simulink model "GuytonModel1972WithSubsystems_R2018_new"  (Simulink 9.1)
settings: Solver=ode23tb  StartTime=0.0  StopTime=inf  RelTol=1e-3  EnableMultiTasking=on
(part 3 of 3)

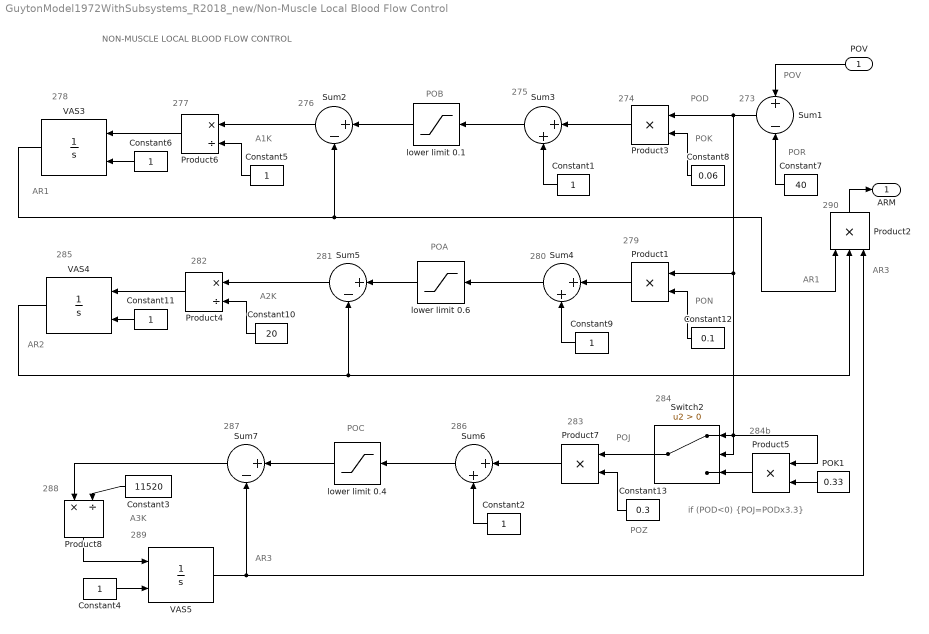
== system GuytonModel1972WithSubsystems_R2018_new/Non-Muscle Local Blood Flow Control  ==
  note: 273
  note: 285
  note: 281
  note: 280
  note: 279
  note: 290
  note: 286
  note: AR2
  note: AR1
  note: 287
  note: AR3
  note: POV
  note: 284b
  note: A2K
  note: POC
  note: AR1
  note: POZ
  note: 284
  note: PON
  note: 288
  note: POR
  note: POJ
  note: 289
  note: POK
  note: POA
  note: NON-MUSCLE LOCAL BLOOD FLOW CONTROL
  note: 278
  note: if (POD<0) {POJ=PODx3.3}
  note: A3K
  note: 282
  note: AR3
  note: 277
  note: 283
  note: 276
  note: 275
  note: POB
  note: 274
  note: A1K
  note: POD
  POV : Inport
  " VAS3" : Integrator  InitialConditionSource=external
  " VAS4" : Integrator  InitialConditionSource=external
  " VAS5" : Integrator  InitialConditionSource=external
  Constant{1..2,4..6,9,11} (7 alike) : Constant
  Constant10 : Constant  Value=20
  Constant12 : Constant  Value=0.1
  Constant13 : Constant  Value=0.3
  Constant3 : Constant  Value=11520
  Constant7 : Constant  Value=40
  Constant8 : Constant  Value=0.06
  POK1 : Constant  Value=0.33
  Product{1,3,5,7} (4 alike) : Product  SaturateOnIntegerOverflow=on  RndMeth=Zero  InputSameDT=on  OutDataTypeStr=Inherit: Same as first input
  Product2 : Product  Inputs=3  SaturateOnIntegerOverflow=on  RndMeth=Zero  InputSameDT=on  OutDataTypeStr=Inherit: Same as first input
  Product4 : Product  Inputs=*/  SaturateOnIntegerOverflow=on  RndMeth=Zero  InputSameDT=on  OutDataTypeStr=Inherit: Same as first input
  Product6 : Product  Inputs=*/  SaturateOnIntegerOverflow=on  RndMeth=Zero  InputSameDT=on  OutDataTypeStr=Inherit: Same as first input
  Product8 : Product  Inputs=*/  SaturateOnIntegerOverflow=on  RndMeth=Zero  InputSameDT=on  OutDataTypeStr=Inherit: Same as first input
  Sum1 : Sum  Inputs=+|-  SaturateOnIntegerOverflow=on  InputSameDT=on  OutDataTypeStr=Inherit: Same as first input
  Sum2 : Sum  Inputs=|+-  SaturateOnIntegerOverflow=on  InputSameDT=on  OutDataTypeStr=Inherit: Same as first input
  Sum3 : Sum  Inputs=|++  SaturateOnIntegerOverflow=on  InputSameDT=on  OutDataTypeStr=Inherit: Same as first input
  Sum4 : Sum  Inputs=|++  SaturateOnIntegerOverflow=on  InputSameDT=on  OutDataTypeStr=Inherit: Same as first input
  Sum5 : Sum  Inputs=|+-  SaturateOnIntegerOverflow=on  InputSameDT=on  OutDataTypeStr=Inherit: Same as first input
  Sum6 : Sum  Inputs=|++  SaturateOnIntegerOverflow=on  InputSameDT=on  OutDataTypeStr=Inherit: Same as first input
  Sum7 : Sum  Inputs=|+-  SaturateOnIntegerOverflow=on  InputSameDT=on  OutDataTypeStr=Inherit: Same as first input
  Switch2 : Switch  Criteria=u2 > Threshold  SaturateOnIntegerOverflow=on  InputSameDT=on
  lower limit 0.1 : Saturate  UpperLimit=inf  LowerLimit=0.2  LinearizeAsGain=off
  lower limit 0.4 : Saturate  UpperLimit=inf  LowerLimit=0.3  LinearizeAsGain=off
  lower limit 0.6 : Saturate  UpperLimit=inf  LowerLimit=0.5  LinearizeAsGain=off
  ARM : Outport
  wires:
  Product2/1 -> ARM/1
  Product7/1 -> Sum6/1
  " VAS3"/1 -> Sum2/2, Product2/1
  lower limit 0.1/1 -> Sum2/1
  Constant3/1 -> Product8/2
  Constant5/1 -> Product6/2
  Product3/1 -> Sum3/1
  Product5/1 -> Switch2/3
  Sum7/1 -> Product8/1
  Product1/1 -> Sum4/1
  POV/1 -> Sum1/1
  " VAS4"/1 -> Sum5/2, Product2/2
  Constant11/1 -> " VAS4"/2
  Constant8/1 -> Product3/2
  Constant10/1 -> Product4/2
  Sum3/1 -> lower limit 0.1/1
  Constant4/1 -> " VAS5"/2
  Product8/1 -> " VAS5"/1
  Product4/1 -> " VAS4"/1
  " VAS5"/1 -> Sum7/2, Product2/3
  POK1/1 -> Product5/2
  Constant6/1 -> " VAS3"/2
  lower limit 0.6/1 -> Sum5/1
  Sum6/1 -> lower limit 0.4/1
  Constant2/1 -> Sum6/2
  Sum5/1 -> Product4/1
  lower limit 0.4/1 -> Sum7/1
  Sum4/1 -> lower limit 0.6/1
  Constant12/1 -> Product1/2
  Constant1/1 -> Sum3/2
  Switch2/1 -> Product7/1
  Constant9/1 -> Sum4/2
  Product6/1 -> " VAS3"/1
  Sum1/1 -> Product3/1, Product1/1, Switch2/1, Product5/1, Switch2/2
  Constant13/1 -> Product7/2
  Sum2/1 -> Product6/1
  Constant7/1 -> Sum1/2

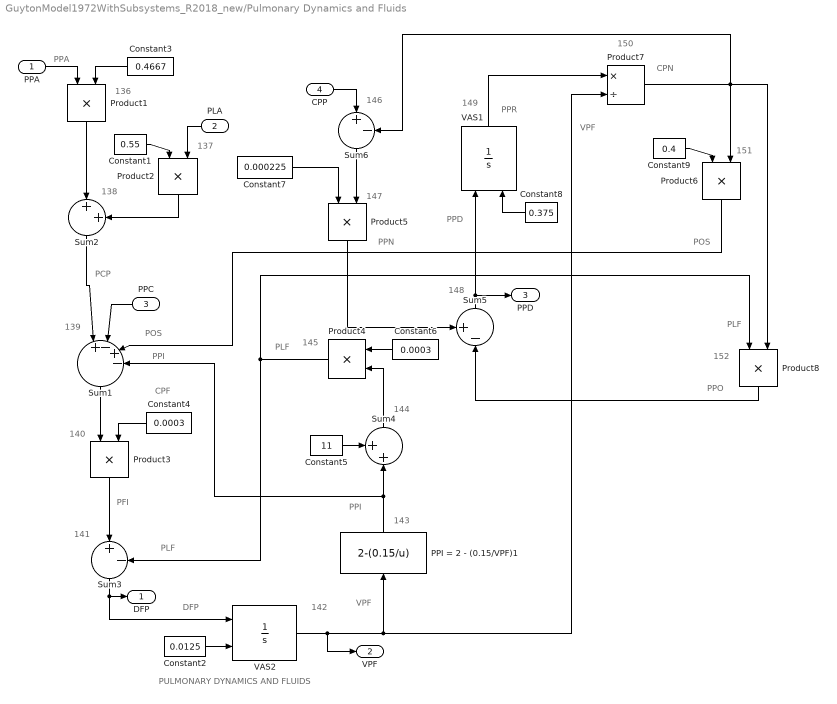
== system GuytonModel1972WithSubsystems_R2018_new/Pulmonary Dynamics and Fluids ==
  note: PULMONARY DYNAMICS AND FLUIDS
  note: 152
  note: 149
  note: 151
  note: POS
  note: DFP
  note: PPR
  note: CPF
  note: PLF
  note: VPF
  note: CPN
  note: VPF
  note: 136
  note: 147
  note: PPN
  note: 137
  note: POS
  note: PPI
  note: PPO
  note: PPD
  note: PLF
  note: PPA
  note: 141
  note: PLF
  note: PCP
  note: 138
  note: 148
  note: PFI
  note: 140
  note: 142
  note: 139
  note: 144
  note: 146
  note: 150
  note: PPI
  note: 143
  note: 145
  PPA : Inport
  PLA : Inport  Port=2
  PPC : Inport  Port=3
  CPP : Inport  Port=4
  " VAS1" : Integrator  InitialConditionSource=external
  " VAS2" : Integrator  InitialConditionSource=external
  Constant1 : Constant  Value=0.55
  Constant2 : Constant  Value=0.0125
  Constant3 : Constant  Value=0.4667
  Constant4 : Constant  Value=0.0003
  Constant5 : Constant  Value=11
  Constant6 : Constant  Value=0.0003
  Constant7 : Constant  Value=0.000225
  Constant8 : Constant  Value=0.375
  Constant9 : Constant  Value=0.4
  PPI = 2 - (0.15/VPF)1 : Fcn  Expr=2-(0.15/u)
  Product{1..6,8} (7 alike) : Product  SaturateOnIntegerOverflow=on  RndMeth=Zero  InputSameDT=on  OutDataTypeStr=Inherit: Same as first input
  Product7 : Product  Inputs=*/  SaturateOnIntegerOverflow=on  RndMeth=Zero  InputSameDT=on  OutDataTypeStr=Inherit: Same as first input
  Sum1 : Sum  Inputs=||+-+-  SaturateOnIntegerOverflow=on  InputSameDT=on  OutDataTypeStr=Inherit: Same as first input
  Sum2 : Sum  Inputs=|++  SaturateOnIntegerOverflow=on  InputSameDT=on  OutDataTypeStr=Inherit: Same as first input
  Sum3 : Sum  Inputs=|+-  SaturateOnIntegerOverflow=on  InputSameDT=on  OutDataTypeStr=Inherit: Same as first input
  Sum4 : Sum  Inputs=++|  SaturateOnIntegerOverflow=on  InputSameDT=on  OutDataTypeStr=Inherit: Same as first input
  Sum5 : Sum  Inputs=+-|  SaturateOnIntegerOverflow=on  InputSameDT=on  OutDataTypeStr=Inherit: Same as first input
  Sum6 : Sum  Inputs=|+-  SaturateOnIntegerOverflow=on  InputSameDT=on  OutDataTypeStr=Inherit: Same as first input
  DFP : Outport
  VPF : Outport  Port=2
  PPD : Outport  Port=3
  wires:
  Constant2/1 -> " VAS2"/2
  Constant3/1 -> Product1/2
  Sum4/1 -> Product4/2
  Sum6/1 -> Product5/2
  Product4/1 -> Product8/1, Sum3/2
  PLA/1 -> Product2/2
  Sum5/1 -> " VAS1"/1, PPD/1
  Constant7/1 -> Product5/1
  Product8/1 -> Sum5/2
  Product5/1 -> Sum5/1
  Sum1/1 -> Product3/1
  Sum2/1 -> Sum1/1
  PPI = 2 - (0.15/VPF)1/1 -> Sum1/4, Sum4/2
  " VAS2"/1 -> VPF/1, PPI = 2 - (0.15/VPF)1/1, Product7/2
  Product6/1 -> Sum1/3
  Constant4/1 -> Product3/2
  Constant6/1 -> Product4/1
  Sum3/1 -> DFP/1, " VAS2"/1
  Constant5/1 -> Sum4/1
  Constant9/1 -> Product6/1
  Product1/1 -> Sum2/1
  PPA/1 -> Product1/1
  Constant1/1 -> Product2/1
  Constant8/1 -> " VAS1"/2
  Product2/1 -> Sum2/2
  " VAS1"/1 -> Product7/1
  Product7/1 -> Product6/2, Sum6/2, Product8/2
  Product3/1 -> Sum3/1
  CPP/1 -> Sum6/1
  PPC/1 -> Sum1/2

== system GuytonModel1972WithSubsystems_R2018_new/Red Cells And Viscosity ==
  note: HKM
  note: 336
  note: HMK
  note: HM
  note: 336b
  note: VIB
  note: HM2
  note: RKC
  note: RED CELLS AND VISCOSITY
  note: 329
  note: HM
  note: PO2
  note: 332
  note: RC1
  note: 330
  note: 331
  note: VRC
  note: VRC
  note: POY
  note: RCD
  note: 334
  note: VIE
  note: RC2
  note: 339
  note: 338
  note: 333
  note: POT
  note: 337
  note: 335
  POT : Inport
  VB : Inport  Port=2
  Constant1 : Constant  Value=464e-7
  Constant133 : Constant  Value=8.25
  Constant2 : Constant  Value=0.0000058
  Constant3 : Constant  Value=100
  Constant5 : Constant  Value=0.5333
  Constant6 : Constant  Value=1.5
  Constant7 : Constant  Value=0.333
  KE 1 : Integrator  InitialConditionSource=external  InitialCondition=74.7024
  Product131 : Product  Inputs=*/  SaturateOnIntegerOverflow=on  RndMeth=Zero  InputSameDT=on  OutDataTypeStr=Inherit: Same as first input
  Product{2..5} (4 alike) : Product  SaturateOnIntegerOverflow=on  RndMeth=Zero  InputSameDT=on  OutDataTypeStr=Inherit: Same as first input
  Product6 : Product  Inputs=*/  SaturateOnIntegerOverflow=on  RndMeth=Zero  InputSameDT=on  OutDataTypeStr=Inherit: Same as first input
  Product7 : Product  Inputs=/*  SaturateOnIntegerOverflow=on  RndMeth=Zero  InputSameDT=on  OutDataTypeStr=Inherit: Same as first input
  Sum101 : Sum  Inputs=+-  SaturateOnIntegerOverflow=on  InputSameDT=on  OutDataTypeStr=Inherit: Same as first input
  Sum2 : Sum  Inputs=+-|  SaturateOnIntegerOverflow=on  InputSameDT=on  OutDataTypeStr=Inherit: Same as first input
  Sum3 : Sum  Inputs=-+|  SaturateOnIntegerOverflow=on  InputSameDT=on  OutDataTypeStr=Inherit: Same as first input
  Sum4 : Sum  Inputs=|++  SaturateOnIntegerOverflow=on  InputSameDT=on  OutDataTypeStr=Inherit: Same as first input
  Z1 : Constant  Value=2
  Z3 : Constant  Value=90
  lower limit 0.2375 : Saturate  UpperLimit=inf  LowerLimit=0.2375  LinearizeAsGain=off
  VIM : Outport
  VRC : Outport  Port=2
  HM : Outport  Port=3
  wires:
  Sum101/1 -> Product131/2
  Z3/1 -> Sum101/1
  Product6/1 -> Product3/2
  Product2/1 -> Sum3/1
  Constant6/1 -> Sum4/1
  POT/1 -> Sum2/2
  Sum3/1 -> KE 1/1
  Constant7/1 -> Product4/1
  Product131/1 -> Product7/2
  Constant2/1 -> Product2/2
  Product5/1 -> Sum3/2
  Product7/1 -> Sum4/2
  Product3/1 -> HM/1, Sum101/2, Product131/1  "HM"
  Sum4/1 -> Product4/2
  Sum2/1 -> lower limit 0.2375/1
  Constant5/1 -> Product7/1
  Constant1/1 -> Product5/2
  Constant3/1 -> Product3/1
  lower limit 0.2375/1 -> Product5/1
  Z1/1 -> KE 1/2
  KE 1/1 -> VRC/1, Product2/1, Product6/1
  VB/1 -> Product6/2  "VB"
  Product4/1 -> VIM/1
  Constant133/1 -> Sum2/1

== system GuytonModel1972WithSubsystems_R2018_new/Thirst And Drinking ==
  note: THIRST AND DRINKING
  note: 190
  note: 194
  note: Z11
  note: Z10
  note: 193
  note: 192
  note: 191
  POT : Inport
  AHM : Inport  Port=2
  Constant1 : Constant  Value=0.01
  Constant2 : Constant  Value=0.009
  Constant3 : Constant  Value=4
  Constant4 : Constant  Value=8.25
  Product1 : Product  SaturateOnIntegerOverflow=on  RndMeth=Zero  InputSameDT=on  OutDataTypeStr=Inherit: Same as first input
  Product2 : Product  SaturateOnIntegerOverflow=on  RndMeth=Zero  InputSameDT=on  OutDataTypeStr=Inherit: Same as first input
  Product3 : Product  SaturateOnIntegerOverflow=on  RndMeth=Zero  InputSameDT=on  OutDataTypeStr=Inherit: Same as first input
  Sum1 : Sum  Inputs=|+-  SaturateOnIntegerOverflow=on  InputSameDT=on  OutDataTypeStr=Inherit: Same as first input
  Sum2 : Sum  Inputs=|-+  SaturateOnIntegerOverflow=on  InputSameDT=on  OutDataTypeStr=Inherit: Same as first input
  lower limit 0 : Saturate  UpperLimit=inf  LowerLimit=0  LinearizeAsGain=off
  STH : Outport
  TVD : Outport  Port=2
  wires:
  lower limit 0/1 -> TVD/1
  POT/1 -> Sum2/1
  Product2/1 -> STH/1, Product1/1
  Product1/1 -> lower limit 0/1
  Sum1/1 -> Product1/2
  Constant2/1 -> Sum1/2
  Product3/1 -> Sum1/1
  Constant1/1 -> Product3/2
  Constant4/1 -> Sum2/2
  Constant3/1 -> Product2/2
  Sum2/1 -> Product2/1
  AHM/1 -> Product3/1

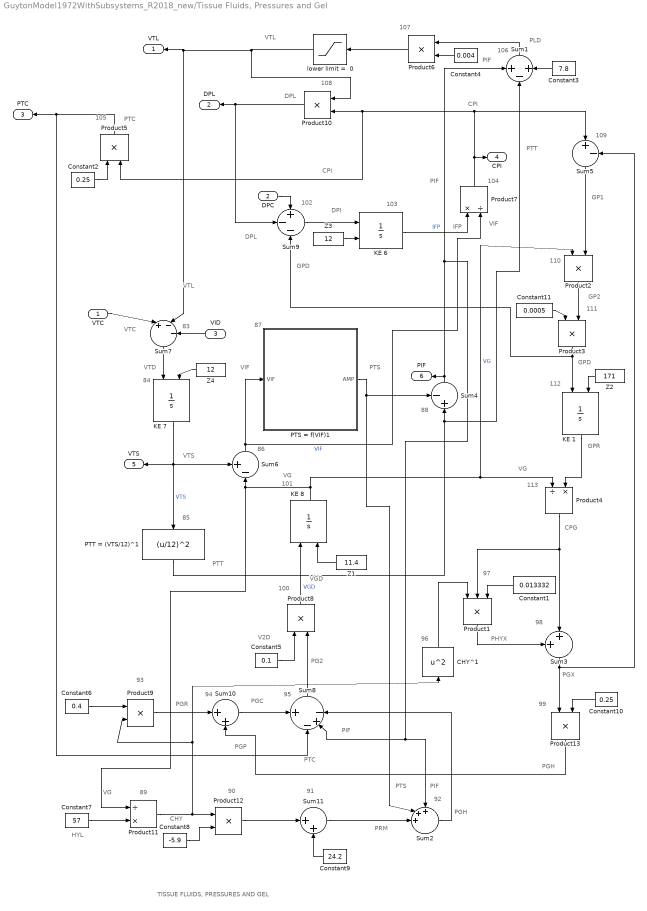
== system GuytonModel1972WithSubsystems_R2018_new/Tissue Fluids, Pressures and Gel ==
  note: CPG
  note: PGX
  note: PHYX
  note: 107
  note: 110
  note: TISSUE FLUIDS, PRESSURES AND GEL
  note: 105
  note: 104
  note: 106
  note: 108
  note: PTC
  note: 109
  note: PTT
  note: 102
  note: CHY
  note: 94
  note: 86
  note: V2D
  note: 84
  note: PTS
  note: VTC
  note: 88
  note: PIF
  note: 89
  note: PTS
  note: PLD
  note: PTT
  note: PGH
  note: VIF
  note: GP2
  note: VGD
  note: HYL
  note: PIF
  note: PTC
  note: VTL
  note: VG
  note: DPI
  note: PGH
  note: 95
  note: 85
  note: VG
  note: 112
  note: 98
  note: CPI
  note: VTL
  note: GPD
  note: DPL
  note: PIF
  note: IFP
  note: VG
  note: GPR
  note: GP1
  note: PGR
  note: 113
  note: 111
  note: 97
  note: 96
  note: 87
  note: 99
  note: 100
  note: VIF
  note: 92
  note: VTD
  note: 101
  note: 83
  note: PGP
  note: PRM
  note: GPD
  note: DPL
  note: 93
  note: 91
  note: PG2
  note: 90
  note: PGC
  note: 103
  note: PIF
  note: VTS
  note: CPI
  VTC : Inport
  DPC : Inport  Port=2
  VID : Inport  Port=3
  CHY^1 : Fcn  Expr=u^2
  Constant1 : Constant  Value=0.013332
  Constant10 : Constant  Value=0.25
  Constant11 : Constant  Value=0.0005
  Constant2 : Constant  Value=0.25
  Constant3 : Constant  Value=7.8
  Constant4 : Constant  Value=0.004
  Constant5 : Constant  Value=0.1
  Constant6 : Constant  Value=0.4
  Constant7 : Constant  Value=57
  Constant8 : Constant  Value=-5.9
  Constant9 : Constant  Value=24.2
  KE {1,6..8} (4 alike) : Integrator  InitialConditionSource=external  InitialCondition=74.7024
  PTS = f(VIF)1 : Subsystem
      mask Display:
      | plot([0    0.5000    1.0000    1.5000    2.0000    2.5000    3.0000    3.5000    4.0000    4.5000    5.0000    5.5000    6.0000    6.5000    7.0000    7.5000    8.0000    8.5000    9.0000    9.5000   10.0000], [19.9974    8.2145    4.9644    3.4422    2.5594    1.9830    1.5771    1.2757    1.0432    0.8583    0.7078    0.5828    0.4775    0.3874    0.3096    0.2416    0.1818    0.1287    0.0812    0.0385   0.0000 ])
      | text(0,22,'')
      | text(0,-2,'')
      | text(-0.5,10,'')
      | text(10.5,10,'')
      | text(-0.2,1,'0')
      | text(0.5,-1,'0')
      | text(-0.2,21,'20')
      | text(9.5,-1,'10')
  PTT = (VTS/12)^1 : Fcn  Expr=(u/12)^2
  Product1 : Product  Inputs=3  SaturateOnIntegerOverflow=on  RndMeth=Zero  InputSameDT=on  OutDataTypeStr=Inherit: Same as first input
  Product{2..3,5..6,8..10,12..13} (9 alike) : Product  SaturateOnIntegerOverflow=on  RndMeth=Zero  InputSameDT=on  OutDataTypeStr=Inherit: Same as first input
  Product11 : Product  Inputs=/*  SaturateOnIntegerOverflow=on  RndMeth=Zero  InputSameDT=on  OutDataTypeStr=Inherit: Same as first input
  Product4 : Product  Inputs=/*  SaturateOnIntegerOverflow=on  RndMeth=Zero  InputSameDT=on  OutDataTypeStr=Inherit: Same as first input
  Product7 : Product  Inputs=*/  SaturateOnIntegerOverflow=on  RndMeth=Zero  InputSameDT=on  OutDataTypeStr=Inherit: Same as first input
  Sum1 : Sum  Inputs=+-+  SaturateOnIntegerOverflow=on  InputSameDT=on  OutDataTypeStr=Inherit: Same as first input
  Sum10 : Sum  Inputs=|++  SaturateOnIntegerOverflow=on  InputSameDT=on  OutDataTypeStr=Inherit: Same as first input
  Sum11 : Sum  Inputs=|++  SaturateOnIntegerOverflow=on  InputSameDT=on  OutDataTypeStr=Inherit: Same as first input
  Sum2 : Sum  Inputs=+++||  SaturateOnIntegerOverflow=on  InputSameDT=on  OutDataTypeStr=Inherit: Same as first input
  Sum3 : Sum  Inputs=++|  SaturateOnIntegerOverflow=on  InputSameDT=on  OutDataTypeStr=Inherit: Same as first input
  Sum4 : Sum  Inputs=-+|  SaturateOnIntegerOverflow=on  InputSameDT=on  OutDataTypeStr=Inherit: Same as first input
  Sum5 : Sum  Inputs=|+-  SaturateOnIntegerOverflow=on  InputSameDT=on  OutDataTypeStr=Inherit: Same as first input
  Sum6 : Sum  Inputs=+-|  SaturateOnIntegerOverflow=on  InputSameDT=on  OutDataTypeStr=Inherit: Same as first input
  Sum7 : Sum  Inputs=|+--  SaturateOnIntegerOverflow=on  InputSameDT=on  OutDataTypeStr=Inherit: Same as first input
  Sum8 : Sum  Inputs=+|-+-  SaturateOnIntegerOverflow=on  InputSameDT=on  OutDataTypeStr=Inherit: Same as first input
  Sum9 : Sum  Inputs=+--  SaturateOnIntegerOverflow=on  InputSameDT=on  OutDataTypeStr=Inherit: Same as first input
  Z1 : Constant  Value=11.4
  Z2 : Constant  Value=171
  Z3 : Constant  Value=12
  Z4 : Constant  Value=12
  lower limit =  0 : Saturate  UpperLimit=inf  LowerLimit=0  LinearizeAsGain=off
  VTL : Outport
  DPL : Outport  Port=2
  PTC : Outport  Port=3
  CPI : Outport  Port=4
  VTS : Outport  Port=5
  PIF : Outport  Port=6
  wires:
  Sum2/1 -> Sum8/4
  Product2/1 -> Product3/2
  Sum9/1 -> KE 6/1
  Product6/1 -> lower limit =  0/1
  Z2/1 -> KE 1/2
  Product4/1 -> Sum3/2, Product1/2
  Z4/1 -> KE 7/2
  Sum8/1 -> Product8/2
  Product1/1 -> Sum3/1
  Constant10/1 -> Product13/2
  Sum7/1 -> KE 7/1
  Product12/1 -> Sum11/1
  Sum3/1 -> Product13/1, Sum5/2
  Constant9/1 -> Sum11/2
  Sum10/1 -> Sum8/1
  PTT = (VTS/12)^1/1 -> Sum4/2, Sum1/2
  Constant5/1 -> Product8/1
  Z1/1 -> KE 8/2
  KE 8/1 -> Sum6/2, Product11/1, Product2/1, Product4/1  "VG"
  Constant8/1 -> Product12/2
  Sum6/1 -> PTS = f(VIF)1/1(VIF), Product7/2  "VIF"
  Constant7/1 -> Product11/2
  CHY^1/1 -> Product1/1
  KE 7/1 -> VTS/1, PTT = (VTS/12)^1/1, Sum6/1  "VTS"
  Constant3/1 -> Sum1/3
  PTS = f(VIF)1/1(AMP) -> Sum2/2, Sum4/1
  VTC/1 -> Sum7/1
  Product5/1 -> PTC/1, Sum8/2
  Sum5/1 -> Product2/2
  Product10/1 -> DPL/1, Sum9/2
  Product13/1 -> Sum10/2
  KE 1/1 -> Product4/2
  Sum4/1 -> Sum2/1, Sum8/3, Sum1/1, PIF/1
  Product3/1 -> Sum9/3, KE 1/1
  Constant11/1 -> Product3/1
  Sum1/1 -> Product6/1
  KE 6/1 -> Product7/1  "IFP"
  Product7/1 -> CPI/1, Product5/2, Product10/2, Sum5/1
  Z3/1 -> KE 6/2
  lower limit =  0/1 -> Sum7/2, VTL/1, Product10/1
  Product11/1 -> Product9/2, CHY^1/1, Product12/1
  Product8/1 -> KE 8/1  "VGD"
  Constant4/1 -> Product6/2
  Constant1/1 -> Product1/3
  Constant6/1 -> Product9/1
  Sum11/1 -> Sum2/3
  Constant2/1 -> Product5/1
  Product9/1 -> Sum10/1
  DPC/1 -> Sum9/1
  VID/1 -> Sum7/3

== system GuytonModel1972WithSubsystems_R2018_new/Vascular Stress Relaxation ==
  note: RVV7
  note: 63
  note: VV1
  note: VV7
  note: VV7
  note: 61
  note: 62
  note: VV2
  note: VV6
  note: SRK
  note: 64
  note: VASCULAR
      | STRESS
      | RELAXATION
  note: VVE
  note: 65
  VVE : Inport
  Constant275 : Constant  Value=0
  Constant32 : Constant  Value=0.301
  Constant33 : Constant  Value=0.5
  Constant34 : Constant  Value=33
  Integrator : Integrator
  Manual Switch58 : ManualSwitch
  Product25 : Product  SaturateOnIntegerOverflow=on  RndMeth=Zero  InputSameDT=on  OutDataTypeStr=Inherit: Same as first input
  Product26 : Product  SaturateOnIntegerOverflow=on  RndMeth=Zero  InputSameDT=on  OutDataTypeStr=Inherit: Same as first input
  Product27 : Product  Inputs=/*  SaturateOnIntegerOverflow=on  RndMeth=Zero  InputSameDT=on  OutDataTypeStr=Inherit: Same as first input
  Sum20 : Sum  Inputs=-+-  SaturateOnIntegerOverflow=on  InputSameDT=on  OutDataTypeStr=Inherit: Same as first input
  VV7 : Outport
  wires:
  Product26/1 -> Sum20/2
  Integrator/1 -> Manual Switch58/1
  Constant275/1 -> Manual Switch58/2
  Constant32/1 -> Product25/1
  Sum20/1 -> Product27/2
  Product25/1 -> Sum20/1
  Manual Switch58/1 -> VV7/1, Sum20/3
  Product27/1 -> Integrator/1
  Constant33/1 -> Product25/2, Product26/1
  Constant34/1 -> Product27/1
  VVE/1 -> Product26/2

== system GuytonModel1972WithSubsystems_R2018_new/Aldosterone Control/AMP = f(PA)1 ==
  PA : Inport
  function StarlingLNorm(PA) cubic spline interpolation x=[0,100,200] y=[4,1,0] : Lookup_n-D  NumberOfTableDimensions=1  BreakpointsForDimension1=[0,100,200]  Table=[4,1,0]  InterpMethod=Cubic spline  ExtrapMethod=Clip  InputSameDT=on
  AMP : Outport
  wires:
  PA/1 -> function StarlingLNorm(PA) cubic spline interpolation x=[0,100,200] y=[4,1,0]/1
  function StarlingLNorm(PA) cubic spline interpolation x=[0,100,200] y=[4,1,0]/1 -> AMP/1

== system GuytonModel1972WithSubsystems_R2018_new/Autonomic Control/AUB calculation1 ==
  note: when PA1<40:            AUB=1.85718
      | when  40>PA1<170:  AUB=0.01426*(170-PA1)
      | when PA1>=170:        AUB=0
  PA1 : Inport
  Constant1 : Constant  Value=170
  Constant2 : Constant  Value=0
  Constant3 : Constant  Value=1.85718
  Gain1 : Gain  Gain=0.014286  SaturateOnIntegerOverflow=on  OutDataTypeStr=Inherit: Same as input  ParamDataTypeStr=Inherit: Same as input
  Sum1 : Sum  Inputs=+-  SaturateOnIntegerOverflow=on  InputSameDT=on  OutDataTypeStr=Inherit: Same as first input
  if (PA1>=170) AUB1=0 else AUB1=0.014286*(80-PA1) : Switch  Threshold=170  SaturateOnIntegerOverflow=on  InputSameDT=on
  "if (PA1>=40) {AUB=AUB1) else AUB=1.859" : Switch  Threshold=40  SaturateOnIntegerOverflow=on  InputSameDT=on
  AUB : Outport  InitialOutput=0
  wires:
  "if (PA1>=40) {AUB=AUB1) else AUB=1.859"/1 -> AUB/1
  Constant3/1 -> "if (PA1>=40) {AUB=AUB1) else AUB=1.859"/3
  if (PA1>=170) AUB1=0 else AUB1=0.014286*(80-PA1)/1 -> "if (PA1>=40) {AUB=AUB1) else AUB=1.859"/1  "AUB1"
  Constant2/1 -> if (PA1>=170) AUB1=0 else AUB1=0.014286*(80-PA1)/1
  Gain1/1 -> if (PA1>=170) AUB1=0 else AUB1=0.014286*(80-PA1)/3
  PA1/1 -> "if (PA1>=40) {AUB=AUB1) else AUB=1.859"/2, if (PA1>=170) AUB1=0 else AUB1=0.014286*(80-PA1)/2, Sum1/2  "PA1"
  Sum1/1 -> Gain1/1
  Constant1/1 -> Sum1/1

== system GuytonModel1972WithSubsystems_R2018_new/Autonomic Control/AUC calculation1 ==
  note: when PA1<40:          AUCC=1.2
      | when  40>PA1<80:  AUC=0.03*(80-PA1)
      | when PA1>=80:        AUC=0
  PA1 : Inport
  Constant1 : Constant  Value=80
  Constant2 : Constant  Value=0
  Constant3 : Constant  Value=1.2
  Gain1 : Gain  Gain=0.03  SaturateOnIntegerOverflow=on  OutDataTypeStr=Inherit: Same as input  ParamDataTypeStr=Inherit: Same as input
  Sum1 : Sum  Inputs=+-  SaturateOnIntegerOverflow=on  InputSameDT=on  OutDataTypeStr=Inherit: Same as first input
  "if (PA1>=40) {AUC=AUC1) else AUC=1.2" : Switch  Threshold=40  SaturateOnIntegerOverflow=on  InputSameDT=on
  if (PA1>=80) AUC1=0 else AUC1=0.03*(80-PA1) : Switch  Threshold=80  SaturateOnIntegerOverflow=on  InputSameDT=on
  AUC : Outport  InitialOutput=0
  wires:
  Constant1/1 -> Sum1/1
  Sum1/1 -> Gain1/1
  PA1/1 -> Sum1/2, if (PA1>=80) AUC1=0 else AUC1=0.03*(80-PA1)/2, "if (PA1>=40) {AUC=AUC1) else AUC=1.2"/2  "PA1"
  Gain1/1 -> if (PA1>=80) AUC1=0 else AUC1=0.03*(80-PA1)/3
  Constant2/1 -> if (PA1>=80) AUC1=0 else AUC1=0.03*(80-PA1)/1
  if (PA1>=80) AUC1=0 else AUC1=0.03*(80-PA1)/1 -> "if (PA1>=40) {AUC=AUC1) else AUC=1.2"/1  "AUC1"
  Constant3/1 -> "if (PA1>=40) {AUC=AUC1) else AUC=1.2"/3
  "if (PA1>=40) {AUC=AUC1) else AUC=1.2"/1 -> AUC/1

== system GuytonModel1972WithSubsystems_R2018_new/Autonomic Control/AUN calculation1 ==
  note: when PA1<20:           AUN=6
      | when  20>PA1<50:  AUN=0.2*(50-PA1)
      | when PA1>=50:        AUN=0
  PA1 : Inport
  Constant1 : Constant  Value=50
  Constant2 : Constant  Value=0
  Constant3 : Constant  Value=6
  Gain1 : Gain  Gain=0.2  SaturateOnIntegerOverflow=on  OutDataTypeStr=Inherit: Same as input  ParamDataTypeStr=Inherit: Same as input
  Sum1 : Sum  Inputs=+-  SaturateOnIntegerOverflow=on  InputSameDT=on  OutDataTypeStr=Inherit: Same as first input
  "if (PA1>=20) {AUN=AUN1) else AUN=6" : Switch  Threshold=20  SaturateOnIntegerOverflow=on  InputSameDT=on
  if (PA1>=50) AUB1=0 else AUN1=0.2*(50-PA1) : Switch  Threshold=50  SaturateOnIntegerOverflow=on  InputSameDT=on
  AUN : Outport  InitialOutput=0
  wires:
  Constant1/1 -> Sum1/1
  Sum1/1 -> Gain1/1
  PA1/1 -> Sum1/2, if (PA1>=50) AUB1=0 else AUN1=0.2*(50-PA1)/2, "if (PA1>=20) {AUN=AUN1) else AUN=6"/2  "PA1"
  Gain1/1 -> if (PA1>=50) AUB1=0 else AUN1=0.2*(50-PA1)/3
  Constant2/1 -> if (PA1>=50) AUB1=0 else AUN1=0.2*(50-PA1)/1
  if (PA1>=50) AUB1=0 else AUN1=0.2*(50-PA1)/1 -> "if (PA1>=20) {AUN=AUN1) else AUN=6"/1  "AUN1"
  Constant3/1 -> "if (PA1>=20) {AUN=AUN1) else AUN=6"/3
  "if (PA1>=20) {AUN=AUN1) else AUN=6"/1 -> AUN/1

== system GuytonModel1972WithSubsystems_R2018_new/Circulatory Dynamics/LVM = f(PA2) ==
  PA2 : Inport
  "function leftHeartLoading(PA2) cubic spline interpolation x=[0,100, 125, 160, 200, 240] y=[1.04, 1.0,0.97,0.88,0.59,0]" : Lookup_n-D  NumberOfTableDimensions=1  BreakpointsForDimension1=[0,70, 100,125, 160, 200, 240]  Table=[1.04, 1.025, 1.0,0.97,0.88,0.59,0]  InterpMethod=Cubic spline  ExtrapMethod=Clip  InputSameDT=on
  LVM : Outport
  wires:
  "function leftHeartLoading(PA2) cubic spline interpolation x=[0,100, 125, 160, 200, 240] y=[1.04, 1.0,0.97,0.88,0.59,0]"/1 -> LVM/1
  PA2/1 -> "function leftHeartLoading(PA2) cubic spline interpolation x=[0,100, 125, 160, 200, 240] y=[1.04, 1.0,0.97,0.88,0.59,0]"/1

== system GuytonModel1972WithSubsystems_R2018_new/Circulatory Dynamics/QLN = f(PLA) ==
  PLA : Inport
  function StarlingLNorm(PLA) cubic spline interpolation x=[-4.5,-4,0,-1,3,6,10] y=[0,0.01,3.6,5.05,9.4,11.6,13.5] : Lookup_n-D  NumberOfTableDimensions=1  BreakpointsForDimension1=[-10,-9,-8,-7,-6,-5,-4.5,-4, -1,0, 3, 6, 10,11,12,13,15]  Table=[0,0,0,0,0,0,0,0.01, 3.6,5.05, 9.4, 11.6,13.5, 13.5, 13.5, 13.5,13.5]  InterpMethod=Cubic spline  ExtrapMethod=Clip  InputSameDT=on
  QLN : Outport
  wires:
  PLA/1 -> function StarlingLNorm(PLA) cubic spline interpolation x=[-4.5,-4,0,-1,3,6,10] y=[0,0.01,3.6,5.05,9.4,11.6,13.5]/1
  function StarlingLNorm(PLA) cubic spline interpolation x=[-4.5,-4,0,-1,3,6,10] y=[0,0.01,3.6,5.05,9.4,11.6,13.5]/1 -> QLN/1

== system GuytonModel1972WithSubsystems_R2018_new/Circulatory Dynamics/QRN = f(PRA) ==
  PRA : Inport
  function StarlingRNorm(PLA) cubic spline interpolation x=[-6,-3,-1,0,2,4,8] y=[0,0.75,2.6,5.0,9.8,12.1,13.5] : Lookup_n-D  NumberOfTableDimensions=1  BreakpointsForDimension1=[-10,-9, -8,-7,-6, -3, -1, 2, 4, 8,8.5, 9,10,11,12,13]  Table=[0,0, 0,0,0,0.75,2.6,9.8,12.1,13.5,13.5,13.5,13.5,13.5,13.5,13.5]  InterpMethod=Cubic spline  ExtrapMethod=Clip  InputSameDT=on
  QRN : Outport
  wires:
  function StarlingRNorm(PLA) cubic spline interpolation x=[-6,-3,-1,0,2,4,8] y=[0,0.75,2.6,5.0,9.8,12.1,13.5]/1 -> QRN/1
  PRA/1 -> function StarlingRNorm(PLA) cubic spline interpolation x=[-6,-3,-1,0,2,4,8] y=[0,0.75,2.6,5.0,9.8,12.1,13.5]/1

== system GuytonModel1972WithSubsystems_R2018_new/Circulatory Dynamics/RVM = f(PP2) ==
  PP2 : Inport
  function rightHeartLoading(PP2) cubic spline interpolation x=[-0,-20,24,30,38,45] y=[1.06,0.97,0.93,0.8,0.46,0] : Lookup_n-D  NumberOfTableDimensions=1  BreakpointsForDimension1=[0,10,20, 24, 30, 38, 45]  Table=[1.06,1.03, 0.97,0.93,0.8,0.46,0]  InterpMethod=Cubic spline  ExtrapMethod=Clip  InputSameDT=on
  RVM : Outport
  wires:
  function rightHeartLoading(PP2) cubic spline interpolation x=[-0,-20,24,30,38,45] y=[1.06,0.97,0.93,0.8,0.46,0]/1 -> RVM/1
  PP2/1 -> function rightHeartLoading(PP2) cubic spline interpolation x=[-0,-20,24,30,38,45] y=[1.06,0.97,0.93,0.8,0.46,0]/1

== system GuytonModel1972WithSubsystems_R2018_new/Tissue Fluids, Pressures and Gel/PTS = f(VIF)1 ==
  VIF : Inport
  Add : Sum
  Add1 : Sum
  Divide : Product  Inputs=*/
  P1 : Gain  Gain=-0.7617
  p2 : Constant  Value=7.617
  q1 : Constant  Value=0.3809
  AMP : Outport
  wires:
  Divide/1 -> AMP/1
  Add/1 -> Divide/1
  Add1/1 -> Divide/2
  q1/1 -> Add1/2
  P1/1 -> Add/1
  p2/1 -> Add/2
  VIF/1 -> Add1/1, P1/1
